simulink model "PCC_Calibration_Simu"  (R2015b)
settings: Solver=ode3  StartTime=0.0  StopTime=1373  FixedStep=0.01  RelTol=1e-3
model workspace: external: MAT-File params.mat (data not in the file)
undefined symbols (not defined in the file): aeroDragCoeff, airDensity, discIntervalf, discIntervals, DiscIntNeverNeededParam, FD, frontArea, G1, G2, G3, G4, G5, G6, gravity, inertialMassVeh, iterNum, lambdaRange, magnitude, massVeh, MDL, powerWeif, powerWeis, predPeriodf, predPeriods, rollingResistCoeff, terminThreshold, terminTimedis, terminVeloweif, terminVeloweis, wheelRadius, z_ACCe
libraries: simulink x16
(part 5 of 5)

== matlab function PCC_Calibration_Simu/Evalution module/MATLAB Function5 ==
  settings: sampleTime=0.01
  data: y1 output; u1 input; u2 input; u3 input; y2 output; u4 input; u5 input; u6 input
function [y1,y2] = fcn(u1,u2,u3,u4,u5,u6)
dis=u1;%单位km
fuel=u2/0.725;%单位L
dis0=u3;%上一时刻的距离
fuel_consumption_acc=u4; %Acc行驶油耗
fuel_saving0=u5;%上一时刻节油率
fuel_avg0=u6;%上一时刻累计油耗
Delta1=0.5;%多出来的续驶里程，间隔2km更新一次
Delta2=0.2;%累计油耗，间隔0.2km更新一次
k_1=fix(dis0/Delta1);
k_2=fix(dis/Delta1);
k1=fix(dis0/Delta2);
k2=fix(dis/Delta2);
%-------------------------------------------------------------------------------计算多出来的续驶里程
if(dis<Delta1)
    B=0;%节油率
else
    if(k_1~=k_2)%开始更新
%         fuel_avg=fuel/dis*100;%pcc平均油耗L/100km
%         fuel_avg_acc=fuel_consumption_acc/dis*100;%acc平均油耗L/100km
        B=(fuel_consumption_acc-fuel_avg0)/fuel_avg0;%与ACC相比，PCC的节油率
    else
        B=fuel_saving0;
    end
end
%-------------------------------------------------------------------------------计算累计油耗
if(dis<Delta2)
    A=4;%平均油耗L/100km
else
    if(k1~=k2)%开始更新
        fuel_avg=fuel/dis*100;%L/100km
        A=fuel_avg;
    else
        A=fuel_avg0;
    end
end
%-------------------------------------------------------------------------------计算结束
y1=round(B*1000)/1000;
y2=round(A*1000)/1000;

== stateflow chart PCC_Calibration_Simu/Subsystem/vehicle_mode/Driveline/FindGear/ShiftLogic ==
  settings: updateMethod=DISCRETE  sampleTime=0.01
  state gear_state [parallel]
    settings: executionOrder=1
    state first
      entry:
      Gear = 1;
      GR = G1;
    state second
      entry:
      Gear = 2;
      GR = G2;
    state third
      entry:
      Gear = 3;
      GR = G3;
    state fourth
      entry:
      Gear = 4;
      GR = G4;
    state fifth
      entry:
      Gear = 5;
      GR = G5;
    state sixth
      entry:
      Gear = 6;
      GR = G6;
    (default) -> first
    second -> third [order 1] : UP
    first -> second : UP
    fourth -> fifth [order 1] : UP
    fifth -> sixth [order 1] : UP
    third -> fourth [order 1] : UP
    third -> second [order 2] : DOWN
    second -> first [order 2] : DOWN
    fifth -> fourth [order 2] : DOWN
    fourth -> third [order 2] : DOWN
    sixth -> fifth : DOWN
  state selection_state [parallel]
    du:[up_th]=calc_up(Gear,APP);
    du:[down_th]=calc_down(Gear,APP);
    settings: executionOrder=2
    state steady_state
    state upshifting
    state downshifting
    (default) -> steady_state
    steady_state -> upshifting [order 1] : [VehicleSpeed > up_th]
    steady_state -> downshifting [order 2] : [VehicleSpeed < down_th && Gear > 1]
    downshifting -> steady_state [order 1] : after(1,tick)
        | [VehicleSpeed <= down_th]
        | {gear_state.DOWN;}
    downshifting -> steady_state [order 2] : [VehicleSpeed > down_th]
    upshifting -> steady_state [order 1] : after(1,tick)
        | [VehicleSpeed >= up_th]
        | {gear_state.UP;}
    upshifting -> steady_state [order 2] : [VehicleSpeed < up_th]
  state up_th = calc_up(Gear,APP) [function]
  state down_th = calc_down(Gear,APP) [function]
  data: Gear function_input; APP function_input; up_th function_output; Gear function_input; APP function_input; down_th function_output; APP input double [0..100]; VehicleSpeed input double; Gear output double; down_th local double; up_th local double; GR output double; G1 parameter double; G2 parameter double; G3 parameter double; G4 parameter double; G5 parameter double; G6 parameter double
  events: DOWN local EITHER_EDGE_EVENT; UP local EITHER_EDGE_EVENT

== matlab function PCC_Calibration_Simu/Subsystem/vehicle_mode/Engine/CalculateEfficiency/MATLAB Function ==
  data: Pout input; eta output; Teng input; Etat input; fmep0 input; fmep1 input; w input; Vdisp input; C2 input
function eta = EngineEfficiency(Pout,Teng,Etat,fmep0,fmep1,w,Vdisp,C2)
%#codegen

eta = Pout/(Pout/(Etat/(1+(fmep0+fmep1*w)/(4*pi*Teng/Vdisp)))+C2*Pout^2);
